simulink model "gm_new_7"  (R2024b)
settings: Solver=FixedStepDiscrete  StartTime=0.0  StopTime=350  RelTol=1e-3
libraries: hdlsllib x6
settings Model: Creator=soumyadeep  LastModifiedBy=soumyadeep
settings OptimizationCC: BlockReduction=off  ConditionallyExecuteInputs=off  DefaultParameterBehavior=Inlined  InheritOutputTypeSmallerThanSingle=on
settings DebuggingCC: AlgebraicLoopMsg=error  InheritedTsInSrcMsg=none  SingleTaskRateTransMsg=error  UnconnectedInputMsg=warning  UnconnectedOutputMsg=warning  UnconnectedLineMsg=warning
settings HardwareCC: ProdBitPerPointer=32  ProdBitPerSizeT=32  ProdBitPerPtrDiffT=32  ProdLargestAtomicFloat=None  ProdIntDivRoundTo=Undefined  ProdEndianess=Unspecified  ProdWordSize=32  ProdHWDeviceType=ASIC/FPGA->ASIC/FPGA  TargetBitPerPointer=64  TargetBitPerSizeT=64  TargetBitPerPtrDiffT=64  TargetLongLongMode=on  TargetIntDivRoundTo=Zero  TargetEndianess=LittleEndian  TargetWordSize=64  TargetHWDeviceType=Custom Processor->MATLAB Host Computer  ProdEqTarget=off

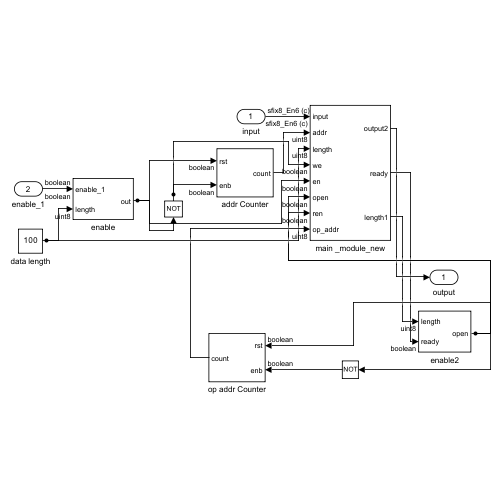
[thumbnail: Simulink's stored preview of the top-level diagram]
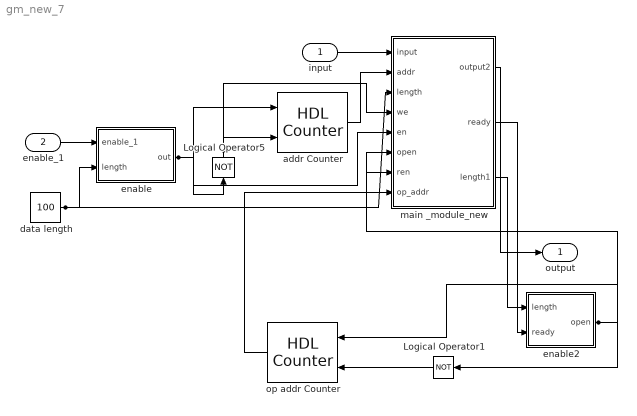
== system gm_new_7 ==
  input : Inport  OutDataTypeStr=fixdt(1, 8, 6)  PortDimensions=1  SampleTime=1
      settings: SignalType=complex
  enable_1 : Inport  Port=2  OutDataTypeStr=boolean  PortDimensions=1  SampleTime=1
  Logical Operator1 : Logic  Operator=NOT  AllPortsSameDT=off  OutDataTypeStr=boolean
  Logical Operator5 : Logic  Operator=NOT  AllPortsSameDT=off  OutDataTypeStr=boolean
  addr Counter : hdlsllib/Sources/HDL Counter  CountType=Count limited  CountInit=0  CountStep=1  CountMax=255  CountFromType=Initial value  CountFrom=0  CountResetPort=on  CountLoadPort=off  CountEnbPort=on  CountDirPort=off  CountHitOutputPort=off  CountDataType=Unsigned  CountWordLen=8  CountFracLen=0  CountSampTime=1
  data length : Constant  Value=100  OutDataTypeStr=uint8  SampleTime=1
  enable : Subsystem
  enable2 : Subsystem
  main _module_new : Subsystem
  op addr Counter : hdlsllib/Sources/HDL Counter  CountType=Count limited  CountInit=0  CountStep=1  CountMax=255  CountFromType=Initial value  CountFrom=0  CountResetPort=on  CountLoadPort=off  CountEnbPort=on  CountDirPort=off  CountHitOutputPort=off  CountDataType=Unsigned  CountWordLen=8  CountFracLen=0  CountSampTime=1
  output : Outport  SampleTime=1
  wires:
  enable_1/1 -> enable/1(enable_1)
  Logical Operator1/1 -> op addr Counter/2
  main _module_new/2(ready) -> enable2/2(ready)
  data length/1 -> main _module_new/3(length), enable/2(length)
  addr Counter/1 -> main _module_new/2(addr)
  enable/1(out) -> Logical Operator5/1, main _module_new/5(en), addr Counter/1
  Logical Operator5/1 -> addr Counter/2, main _module_new/4(we)
  op addr Counter/1 -> main _module_new/8(op_addr)
  input/1 -> main _module_new/1(input)
  enable2/1(open) -> main _module_new/6(open), op addr Counter/1, main _module_new/7(ren), Logical Operator1/1
  main _module_new/1(output2) -> output/1
  main _module_new/3(length1) -> enable2/1(length)

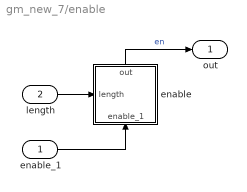
== system gm_new_7/enable ==
  enable_1 : Inport  OutDataTypeStr=boolean  PortDimensions=1  SampleTime=1
  length : Inport  Port=2  OutDataTypeStr=uint8  PortDimensions=1  SampleTime=1
  enable : Stateflow chart  TreatAsAtomicUnit=on
      settings: PortSchema="{\"entries\":[{\"content\":{\"sides\":[{\"content\":{\"connectorIds\":[\"In2\"]},\"type\":\"ConnectorPlacement.EquallySpacedRectSide\",\"uuid\":\"d4f734a1-5378-4a5e-bf96-9f30f80742a7\"},{\"content\":{\"side\":\"RIGHT\"},\"type\":\"ConnectorPlacement.EquallySpacedRectSide\",\"uuid\":\"fbe0227d-1575-4e50-a04f-160a74c8536d\"},{\"content\":{\"connectorIds\":[\"Out1\"],\"side\":\"TOP\"},\"type\":\"ConnectorPlacement.EquallySpacedRectSide\",\"uuid\":\"6983a355-c03c-4e79-af5c-7538764b1859\"},{\"content\":{\"connectorIds\":[\"In1\"],\"side\":\"BOTTOM\"},\"type\":\"ConnectorPlacement.EquallySpacedRectSide\",\"uuid\":\"dc3d3e37-a8de-426f-896b-987f371124ff\"}]},\"type\":\"ConnectorPlacement.EquallySpacedConnector\",\"uuid\":\"0727d717-0168-4707-98f4-9f4fe999d9ac\"}],\"packageUris\":[\"http://schema.mathworks.com/mf0/Connector/R2020b\"],\"version\":\"1.0\"}"
  out : Outport  SampleTime=1
  wires:
  enable/1(out) -> out/1  "en"
  length/1 -> enable/2(length)
  enable_1/1 -> enable/1(enable_1)

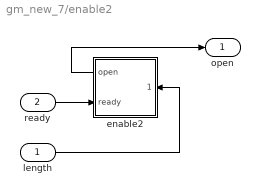
== system gm_new_7/enable2 ==
  length : Inport  OutDataTypeStr=uint8  PortDimensions=1  SampleTime=1
  ready : Inport  Port=2  OutDataTypeStr=boolean  PortDimensions=1  SampleTime=1
  enable2 : Stateflow chart  TreatAsAtomicUnit=on
      settings: PortSchema="{\"entries\":[{\"content\":{\"sides\":[{\"content\":{\"connectorIds\":[\"Out1\",\"In2\"]},\"type\":\"ConnectorPlacement.EquallySpacedRectSide\",\"uuid\":\"e976b215-c191-4a2d-ab29-ab840cb269e6\"},{\"content\":{\"connectorIds\":[\"In1\"],\"side\":\"RIGHT\"},\"type\":\"ConnectorPlacement.EquallySpacedRectSide\",\"uuid\":\"2babecd7-8985-4569-9a06-cece2b2ffb8f\"},{\"content\":{\"side\":\"TOP\"},\"type\":\"ConnectorPlacement.EquallySpacedRectSide\",\"uuid\":\"af427235-ee93-482e-9756-aec73c72c9f8\"}]},\"type\":\"ConnectorPlacement.EquallySpacedConnector\",\"uuid\":\"44840770-11b5-4ed5-8fb6-b77eafe90a2c\"}],\"packageUris\":[\"http://schema.mathworks.com/mf0/Connector/R2020b\"],\"version\":\"1.0\"}"
  open : Outport  SampleTime=1
  wires:
  ready/1 -> enable2/2(ready)
  length/1 -> enable2/1(length)
  enable2/1(open) -> open/1

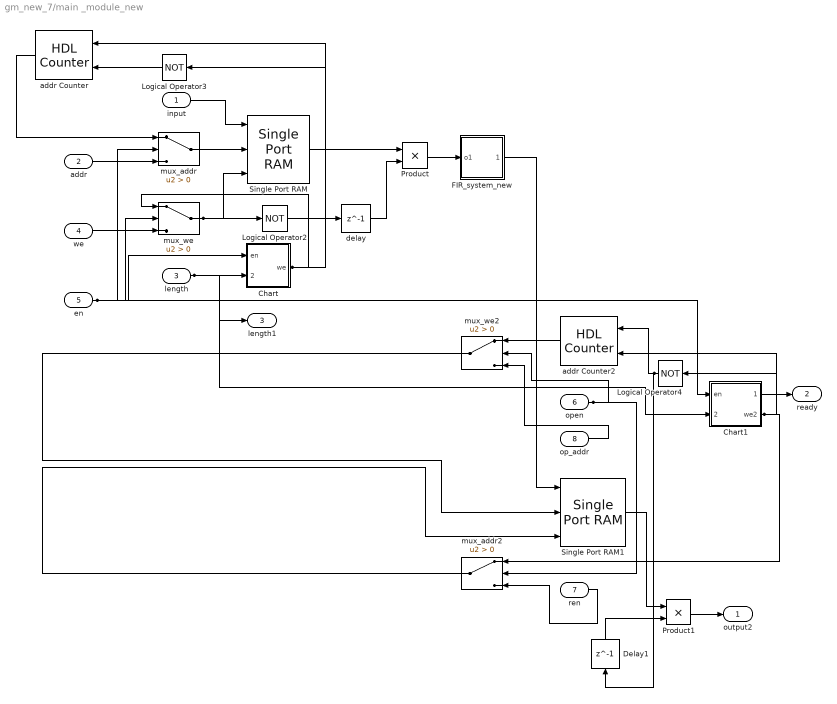
== system gm_new_7/main _module_new ==
  input : Inport  OutDataTypeStr=fixdt(1, 8, 6)  PortDimensions=1  SampleTime=1
      settings: SignalType=complex
  addr : Inport  Port=2  OutDataTypeStr=uint8  PortDimensions=1  SampleTime=1
  length : Inport  Port=3  OutDataTypeStr=uint8  PortDimensions=1  SampleTime=1
  we : Inport  Port=4  OutDataTypeStr=boolean  PortDimensions=1  SampleTime=1
  en : Inport  Port=5  OutDataTypeStr=boolean  PortDimensions=1  SampleTime=1
  open : Inport  Port=6  OutDataTypeStr=boolean  PortDimensions=1  SampleTime=1
  ren : Inport  Port=7  OutDataTypeStr=boolean  PortDimensions=1  SampleTime=1
  op_addr : Inport  Port=8  OutDataTypeStr=uint8  PortDimensions=1  SampleTime=1
  Chart : Subsystem
  Chart1 : Subsystem
  Delay1 : Delay  DelayLength=1  InitialCondition=0  SampleTime=1
  FIR_system_new : Subsystem
  Logical Operator2 : Logic  Operator=NOT  AllPortsSameDT=off  OutDataTypeStr=boolean
  Logical Operator3 : Logic  Operator=NOT  AllPortsSameDT=off  OutDataTypeStr=boolean
  Logical Operator4 : Logic  Operator=NOT  AllPortsSameDT=off  OutDataTypeStr=boolean
  Product : Product  OutDataTypeStr=fixdt(1,8,6)
  Product1 : Product  OutDataTypeStr=fixdt(1,8,6)
  Single Port RAM : hdlsllib/HDL RAMs/Single Port RAM  ram_size=8  dout_type=New data
  Single Port RAM1 : hdlsllib/HDL RAMs/Single Port RAM  ram_size=8  dout_type=New data
  addr Counter : hdlsllib/Sources/HDL Counter  CountType=Count limited  CountInit=0  CountStep=1  CountMax=255  CountFromType=Initial value  CountFrom=0  CountResetPort=on  CountLoadPort=off  CountEnbPort=on  CountDirPort=off  CountHitOutputPort=off  CountDataType=Unsigned  CountWordLen=8  CountFracLen=0  CountSampTime=1
  addr Counter2 : hdlsllib/Sources/HDL Counter  CountType=Count limited  CountInit=0  CountStep=1  CountMax=255  CountFromType=Initial value  CountFrom=0  CountResetPort=on  CountLoadPort=off  CountEnbPort=on  CountDirPort=off  CountHitOutputPort=off  CountDataType=Unsigned  CountWordLen=8  CountFracLen=0  CountSampTime=1
  delay : Delay  DelayLength=1  InitialCondition=0  SampleTime=1
  mux_addr : Switch  Criteria=u2 > Threshold  OutDataTypeStr=uint8  SaturateOnIntegerOverflow=off  InputSameDT=off
  mux_addr2 : Switch  Criteria=u2 > Threshold  OutDataTypeStr=boolean  SaturateOnIntegerOverflow=off  InputSameDT=off
  mux_we : Switch  Criteria=u2 > Threshold  OutDataTypeStr=boolean  SaturateOnIntegerOverflow=off  InputSameDT=off
  mux_we2 : Switch  Criteria=u2 > Threshold  OutDataTypeStr=uint8  SaturateOnIntegerOverflow=off  InputSameDT=off
  output2 : Outport  SampleTime=1
  ready : Outport  Port=2  SampleTime=1
  length1 : Outport  Port=3  SampleTime=1
  wires:
  length/1 -> Chart1/2(length), Chart/2(length), length1/1
  addr Counter/1 -> mux_addr/1
  Chart1/2(we2) -> Logical Operator4/1, addr Counter2/2, mux_addr2/1
  mux_we/1 -> Logical Operator2/1, Single Port RAM/3
  addr/1 -> mux_addr/3
  delay/1 -> Product/2
  Logical Operator2/1 -> delay/1
  we/1 -> mux_we/3
  mux_addr/1 -> Single Port RAM/2
  en/1 -> Chart1/1(en), Chart/1(en), mux_we/2, mux_addr/2
  Logical Operator3/1 -> addr Counter/2
  Delay1/1 -> Product1/2
  input/1 -> Single Port RAM/1
  Single Port RAM/1 -> Product/1
  Chart/1(we) -> mux_we/1, addr Counter/1, Logical Operator3/1
  Product/1 -> FIR_system_new/1(o1)
  mux_we2/1 -> Single Port RAM1/2
  mux_addr2/1 -> Single Port RAM1/3
  FIR_system_new/1(output) -> Single Port RAM1/1
  addr Counter2/1 -> mux_we2/1
  open/1 -> mux_we2/2, mux_addr2/2
  op_addr/1 -> mux_we2/3
  Single Port RAM1/1 -> Product1/1
  ren/1 -> mux_addr2/3
  Logical Operator4/1 -> Delay1/1, addr Counter2/1
  Product1/1 -> output2/1
  Chart1/1(ready) -> ready/1

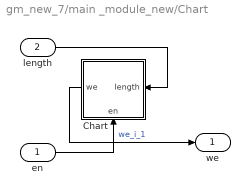
== system gm_new_7/main _module_new/Chart ==
  en : Inport  OutDataTypeStr=boolean  PortDimensions=1  SampleTime=1
  length : Inport  Port=2  OutDataTypeStr=uint8  PortDimensions=1  SampleTime=1
  Chart : Stateflow chart  TreatAsAtomicUnit=on
      settings: PortSchema="{\"entries\":[{\"content\":{\"sides\":[{\"content\":{\"connectorIds\":[\"In2\"]},\"type\":\"ConnectorPlacement.EquallySpacedRectSide\",\"uuid\":\"9d26f323-fb28-4001-b1d4-937ed83cbce6\"},{\"content\":{\"connectorIds\":[\"Out1\"],\"side\":\"RIGHT\"},\"type\":\"ConnectorPlacement.EquallySpacedRectSide\",\"uuid\":\"67176339-3546-49aa-b02e-48370b74535f\"},{\"content\":{\"side\":\"TOP\"},\"type\":\"ConnectorPlacement.EquallySpacedRectSide\",\"uuid\":\"7184d725-8678-4718-ab18-dc31a61fdf5b\"},{\"content\":{\"connectorIds\":[\"In1\"],\"side\":\"BOTTOM\"},\"type\":\"ConnectorPlacement.EquallySpacedRectSide\",\"uuid\":\"e76eb572-4d55-4d8c-bbc9-2fa24e3a43b1\"}]},\"type\":\"ConnectorPlacement.EquallySpacedConnector\",\"uuid\":\"0f16bf70-e106-446b-a3e1-c4bb6d380e54\"}],\"packageUris\":[\"http://schema.mathworks.com/mf0/Connector/R2020b\"],\"version\":\"1.0\"}"
  we : Outport  SampleTime=1
  wires:
  length/1 -> Chart/2(length)
  en/1 -> Chart/1(en)
  Chart/1(we) -> we/1  "we_i_1"

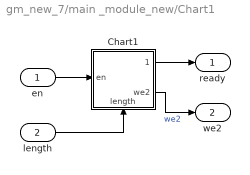
== system gm_new_7/main _module_new/Chart1 ==
  en : Inport  OutDataTypeStr=boolean  PortDimensions=1  SampleTime=1
  length : Inport  Port=2  OutDataTypeStr=uint8  PortDimensions=1  SampleTime=1
  Chart1 : Stateflow chart  TreatAsAtomicUnit=on
      settings: PortSchema="{\"entries\":[{\"content\":{\"sides\":[{\"content\":{\"connectorIds\":[\"In1\"]},\"type\":\"ConnectorPlacement.EquallySpacedRectSide\",\"uuid\":\"9d26f323-fb28-4001-b1d4-937ed83cbce6\"},{\"content\":{\"connectorIds\":[\"Out1\",\"Out2\"],\"side\":\"RIGHT\"},\"type\":\"ConnectorPlacement.EquallySpacedRectSide\",\"uuid\":\"67176339-3546-49aa-b02e-48370b74535f\"},{\"content\":{\"side\":\"TOP\"},\"type\":\"ConnectorPlacement.EquallySpacedRectSide\",\"uuid\":\"7184d725-8678-4718-ab18-dc31a61fdf5b\"},{\"content\":{\"connectorIds\":[\"In2\"],\"side\":\"BOTTOM\"},\"type\":\"ConnectorPlacement.EquallySpacedRectSide\",\"uuid\":\"e76eb572-4d55-4d8c-bbc9-2fa24e3a43b1\"}]},\"type\":\"ConnectorPlacement.EquallySpacedConnector\",\"uuid\":\"0f16bf70-e106-446b-a3e1-c4bb6d380e54\"}],\"packageUris\":[\"http://schema.mathworks.com/mf0/Connector/R2020b\"],\"version\":\"1.0\"}"
  ready : Outport  SampleTime=1
  we2 : Outport  Port=2  SampleTime=1
  wires:
  en/1 -> Chart1/1(en)
  length/1 -> Chart1/2(length)
  Chart1/1(ready) -> ready/1
  Chart1/2(we2) -> we2/1  "we2"

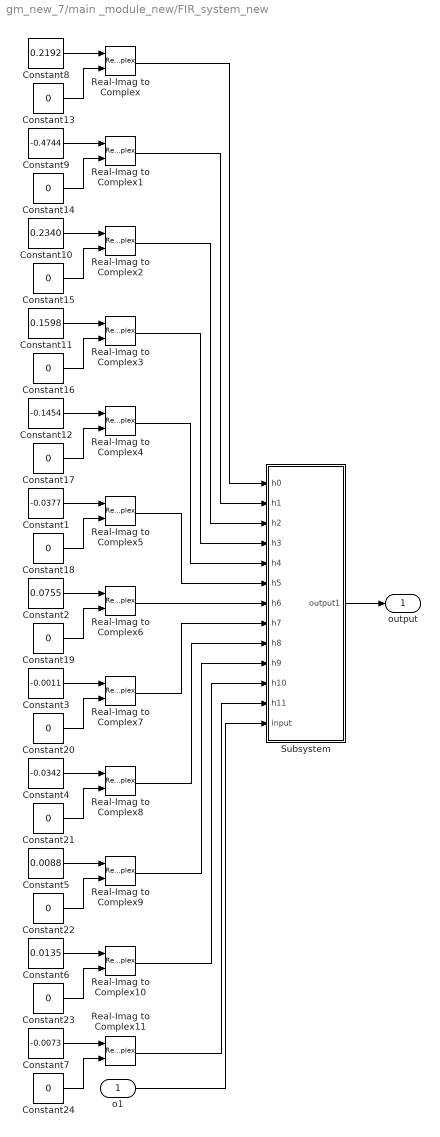
== system gm_new_7/main _module_new/FIR_system_new ==
  o1 : Inport  OutDataTypeStr=fixdt(1, 8, 6)  PortDimensions=1  SampleTime=1
      settings: SignalType=complex
  Constant1 : Constant  Value=-0.0377  OutDataTypeStr=fixdt(1,8,6)  SampleTime=1
  Constant10 : Constant  Value=0.2340  OutDataTypeStr=fixdt(1,8,6)  SampleTime=1
  Constant11 : Constant  Value=0.1598  OutDataTypeStr=fixdt(1,8,6)  SampleTime=1
  Constant12 : Constant  Value=-0.1454  OutDataTypeStr=fixdt(1,8,6)  SampleTime=1
  Constant{13..24} (12 alike) : Constant  Value=0  OutDataTypeStr=fixdt(1,8,6)  SampleTime=1
  Constant2 : Constant  Value=0.0755  OutDataTypeStr=fixdt(1,8,6)  SampleTime=1
  Constant3 : Constant  Value=-0.0011  OutDataTypeStr=fixdt(1,8,6)  SampleTime=1
  Constant4 : Constant  Value=-0.0342  OutDataTypeStr=fixdt(1,8,6)  SampleTime=1
  Constant5 : Constant  Value=0.0088  OutDataTypeStr=fixdt(1,8,6)  SampleTime=1
  Constant6 : Constant  Value=0.0135  OutDataTypeStr=fixdt(1,8,6)  SampleTime=1
  Constant7 : Constant  Value=-0.0073  OutDataTypeStr=fixdt(1,8,6)  SampleTime=1
  Constant8 : Constant  Value=0.2192  OutDataTypeStr=fixdt(1,8,6)  SampleTime=1
  Constant9 : Constant  Value=-0.4744  OutDataTypeStr=fixdt(1,8,6)  SampleTime=1
  Real-Imag to Complex{,1..11} (12 alike) : RealImagToComplex
  Subsystem : Subsystem
  output : Outport  SampleTime=1
  wires:
  Constant15/1 -> Real-Imag to Complex2/2
  Constant8/1 -> Real-Imag to Complex/1
  Constant13/1 -> Real-Imag to Complex/2
  Constant9/1 -> Real-Imag to Complex1/1
  Real-Imag to Complex2/1 -> Subsystem/3(h2)
  Constant14/1 -> Real-Imag to Complex1/2
  Constant10/1 -> Real-Imag to Complex2/1
  Constant11/1 -> Real-Imag to Complex3/1
  Constant16/1 -> Real-Imag to Complex3/2
  Constant12/1 -> Real-Imag to Complex4/1
  Constant17/1 -> Real-Imag to Complex4/2
  o1/1 -> Subsystem/13(input)
  Constant1/1 -> Real-Imag to Complex5/1
  Real-Imag to Complex8/1 -> Subsystem/9(h8)
  Constant18/1 -> Real-Imag to Complex5/2
  Real-Imag to Complex5/1 -> Subsystem/6(h5)
  Constant2/1 -> Real-Imag to Complex6/1
  Constant19/1 -> Real-Imag to Complex6/2
  Constant3/1 -> Real-Imag to Complex7/1
  Constant20/1 -> Real-Imag to Complex7/2
  Constant4/1 -> Real-Imag to Complex8/1
  Constant21/1 -> Real-Imag to Complex8/2
  Constant5/1 -> Real-Imag to Complex9/1
  Constant22/1 -> Real-Imag to Complex9/2
  Constant6/1 -> Real-Imag to Complex10/1
  Constant23/1 -> Real-Imag to Complex10/2
  Constant7/1 -> Real-Imag to Complex11/1
  Constant24/1 -> Real-Imag to Complex11/2
  Real-Imag to Complex4/1 -> Subsystem/5(h4)
  Real-Imag to Complex/1 -> Subsystem/1(h0)
  Real-Imag to Complex1/1 -> Subsystem/2(h1)
  Real-Imag to Complex3/1 -> Subsystem/4(h3)
  Real-Imag to Complex6/1 -> Subsystem/7(h6)
  Real-Imag to Complex7/1 -> Subsystem/8(h7)
  Real-Imag to Complex9/1 -> Subsystem/10(h9)
  Real-Imag to Complex10/1 -> Subsystem/11(h10)
  Real-Imag to Complex11/1 -> Subsystem/12(h11)
  Subsystem/1(output1) -> output/1

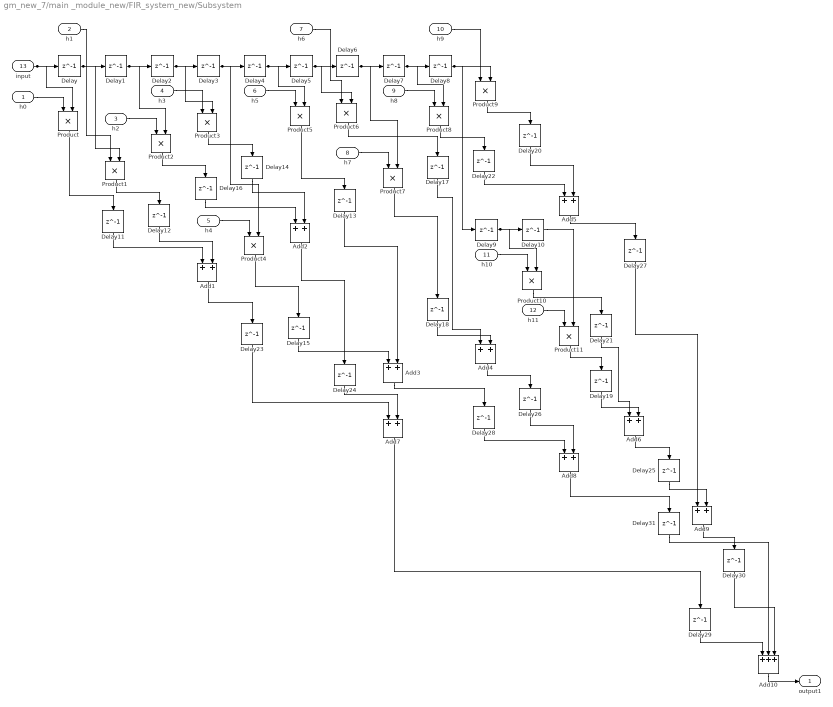
== system gm_new_7/main _module_new/FIR_system_new/Subsystem ==
  h0 : Inport  OutDataTypeStr=fixdt(1, 8, 6)  PortDimensions=1  SampleTime=1
      settings: SignalType=complex
  h1 : Inport  Port=2  OutDataTypeStr=fixdt(1, 8, 6)  PortDimensions=1  SampleTime=1
      settings: SignalType=complex
  h2 : Inport  Port=3  OutDataTypeStr=fixdt(1, 8, 6)  PortDimensions=1  SampleTime=1
      settings: SignalType=complex
  h3 : Inport  Port=4  OutDataTypeStr=fixdt(1, 8, 6)  PortDimensions=1  SampleTime=1
      settings: SignalType=complex
  h4 : Inport  Port=5  OutDataTypeStr=fixdt(1, 8, 6)  PortDimensions=1  SampleTime=1
      settings: SignalType=complex
  h5 : Inport  Port=6  OutDataTypeStr=fixdt(1, 8, 6)  PortDimensions=1  SampleTime=1
      settings: SignalType=complex
  h6 : Inport  Port=7  OutDataTypeStr=fixdt(1, 8, 6)  PortDimensions=1  SampleTime=1
      settings: SignalType=complex
  h7 : Inport  Port=8  OutDataTypeStr=fixdt(1, 8, 6)  PortDimensions=1  SampleTime=1
      settings: SignalType=complex
  h8 : Inport  Port=9  OutDataTypeStr=fixdt(1, 8, 6)  PortDimensions=1  SampleTime=1
      settings: SignalType=complex
  h9 : Inport  Port=10  OutDataTypeStr=fixdt(1, 8, 6)  PortDimensions=1  SampleTime=1
      settings: SignalType=complex
  h10 : Inport  Port=11  OutDataTypeStr=fixdt(1, 8, 6)  PortDimensions=1  SampleTime=1
      settings: SignalType=complex
  h11 : Inport  Port=12  OutDataTypeStr=fixdt(1, 8, 6)  PortDimensions=1  SampleTime=1
      settings: SignalType=complex
  input : Inport  Port=13  OutDataTypeStr=fixdt(1, 8, 6)  PortDimensions=1  SampleTime=1
      settings: SignalType=complex
  Add1 : Sum  OutDataTypeStr=fixdt(1,8,6)
  Add10 : Sum  Inputs=+++  OutDataTypeStr=fixdt(1, 8, 6)  AccumDataTypeStr=fixdt(1,8,6)
  Add2 : Sum  OutDataTypeStr=fixdt(1,8,6)
  Add{3..7} (5 alike) : Sum  OutDataTypeStr=fixdt(1, 9, 6)
  Add8 : Sum  OutDataTypeStr=fixdt(1, 10, 6)
  Add9 : Sum  OutDataTypeStr=fixdt(1, 10, 6)
  Delay{,1..31} (32 alike) : Delay  DelayLength=1  InitialCondition=0  SampleTime=1
  Product{,1..11} (12 alike) : Product  OutDataTypeStr=fixdt(1,8,6)
  output1 : Outport  OutDataTypeStr=fixdt(1,8,6)  SampleTime=1  VectorParamsAs1DForOutWhenUnconnected=off
  wires:
  Product8/1 -> Delay22/1
  Delay11/1 -> Add1/1
  Product4/1 -> Delay15/1
  input/1 -> Product/2, Delay/1
  Delay31/1 -> Add10/2
  h0/1 -> Product/1
  Product6/1 -> Delay17/1
  Delay/1 -> Product1/2, Delay1/1
  Product/1 -> Delay11/1
  h1/1 -> Product1/1
  h5/1 -> Product5/1
  Product1/1 -> Delay12/1
  Delay1/1 -> Product2/2, Delay2/1
  Delay2/1 -> Product3/2, Delay3/1
  h2/1 -> Product2/1
  h9/1 -> Product9/1
  Product2/1 -> Delay16/1
  Product9/1 -> Delay20/1
  Delay12/1 -> Add1/2
  h3/1 -> Product3/1
  Product3/1 -> Delay14/1
  Delay16/1 -> Add2/1
  Add1/1 -> Delay23/1
  Delay3/1 -> Product4/2, Delay4/1
  h4/1 -> Product4/1
  Delay14/1 -> Add2/2
  Delay23/1 -> Add7/1
  Delay4/1 -> Product5/2, Delay5/1
  Product5/1 -> Delay13/1
  Delay17/1 -> Add4/1
  Add2/1 -> Delay24/1
  Delay15/1 -> Add3/1
  h6/1 -> Product6/1
  Delay5/1 -> Product6/2, Delay6/1
  Delay13/1 -> Add3/2
  Add8/1 -> Delay31/1
  Delay24/1 -> Add7/2
  Delay6/1 -> Product7/2, Delay7/1
  h7/1 -> Product7/1
  Product7/1 -> Delay18/1
  Delay18/1 -> Add4/2
  Add3/1 -> Delay28/1
  Add7/1 -> Delay29/1
  Delay7/1 -> Delay8/1, Product8/2
  Product11/1 -> Delay19/1
  h8/1 -> Product8/1
  Delay8/1 -> Delay9/1, Product9/2
  Delay22/1 -> Add5/1
  Add4/1 -> Delay26/1
  Delay28/1 -> Add8/1
  Delay9/1 -> Product10/2, Delay10/1
  h10/1 -> Product10/1
  Add5/1 -> Delay27/1
  Delay20/1 -> Add5/2
  Product10/1 -> Delay21/1
  Delay26/1 -> Add8/2
  Delay10/1 -> Product11/2
  h11/1 -> Product11/1
  Add6/1 -> Delay25/1
  Delay21/1 -> Add6/1
  Delay19/1 -> Add6/2
  Delay27/1 -> Add9/1
  Add9/1 -> Delay30/1
  Delay25/1 -> Add9/2
  Delay29/1 -> Add10/1
  Delay30/1 -> Add10/3
  Add10/1 -> output1/1

== stateflow chart gm_new_7/main _module_new/Chart1/Chart1 ==
  settings: updateMethod=DISCRETE  sampleTime=1  executeAtInitialization=1
  state nop
    entry:
    we2=false;
    i2=0
  state nop3
    entry:
    we2=false;
    ready=true;
  state nop2
    entry:
    we2=false;
    i2=i2+1;
  state write
    entry:
    we2=true;
    i2=i2+1;
  (default) -> nop
  nop -> nop [order 1] : [en==0]
  nop3 -> nop : [en==0]
  nop -> nop2 [order 2] : [en==1]
  write -> nop3 [order 2] : [i2==4+length+12-1]
  write -> write [order 1] : [i2<4+length+12-1]
  nop2 -> nop2 [order 2] : [i2<4]
  nop2 -> write [order 1] : [i2==4]
  data: ready output boolean; we2 output boolean; en input boolean; length input uint8; i2 local uint8

== stateflow chart gm_new_7/enable2/enable2 ==
  settings: executeAtInitialization=1
  state opread
    entry:
    open=false;
    i=i+1;
  state nop1
    entry:
    open=true;
    i=0
  state nop2
    entry:
    open=true;
    i=0
  (default) -> nop1
  nop1 -> opread [order 1] : [ready==1]
  opread -> opread [order 1] : [i<length+12-1]
  nop1 -> nop1 [order 2] : [ready==0]
  nop2 -> nop1 : [ready==0]
  opread -> nop2 [order 2] : [i==length+12-1]
  data: length input uint8; i local uint8 =0; ready input boolean; open output boolean

== stateflow chart gm_new_7/enable/enable ==
  settings: updateMethod=DISCRETE  sampleTime=1  executeAtInitialization=1
  state nop0
  state S0
    entry:
    i=i+1;
  state nop
    entry:
    out =~out;
  (default) -> nop0
  nop0 -> S0 [order 1] : [enable_1==1]
  nop0 -> nop0 [order 2] : [enable_1==0]
  S0 -> nop [order 1] : [i==length]
  S0 -> S0 [order 2] : [i<length]
  data: enable_1 input boolean; out output boolean =0; i local uint8 =0; length input

== stateflow chart gm_new_7/main _module_new/Chart/Chart ==
  settings: updateMethod=DISCRETE  sampleTime=1  executeAtInitialization=1
  state nop2
    entry:
    we=true;
  state nop
    entry:
    we=true;
    i1=0
  state read
    entry:
    we=false;
    i1=i1+1;
  (default) -> nop
  nop -> nop [order 1] : [en==0]
  nop2 -> nop : [en==0]
  nop -> read [order 2] : [en==1]
  read -> nop2 [order 2] : [i1==length]
  read -> read [order 1] : [i1<length]
  data: we output boolean =1; en input boolean; length input uint8; i1 local uint8
